simulink model "YCbCrTesting"  (Simulink 7.7)
settings: Solver=ode45  StartTime=0.0  StopTime=10.0  RelTol=1e-3
undefined symbols (not defined in the file or in its folder): gray, M, N, Rec, SDTV, sz
libraries: vipmisc x22, dspsigops x7, viptransforms x6, viputilities x6, vipconversions x4, dspobslib x4, vipobslib x1, dspsrcs4 x1, vipsnks x1
(part 2 of 2)

== matlab function Decoder/Block Processing/Block iterator/sub-block process/Transform decoder1/Bit Unpack ==
  data: in input double; out output single size=64
function out=bitunpack(in)

% Unpack the bits packed by the bit pack block. If there are not enough 
% values in the packed stream the rest of the output is filled with zeros.

persistent prev_out;
if isempty(prev_out)
    prev_out = single(zeros(64,1));
end
    out = prev_out;
    cbits= int32(0); 
    inpos=2; 
    Temp = uint32(0); 
    run = uint32(0);
    val = uint32(0);
   
    numcoefs = 64;
    if bitget(in(1),32)%negative
        out(1)=-int32(intmax('uint32')- uint32(in(1))) - int32(1);
    else
        out(1)=int32(in(1));
    end
    
    % ac coefficients
    % 4 bit - run length followed by 8 bit coef value  
    i=2;
    while (i<=numcoefs)   
         
        [flag, cbits, inpos, Temp, run] = getbits(cbits, inpos, Temp, in, run, 4);
        if (~flag) 
            break; 
        end
        if (run == 15), break;   end % end of stream  
        
        [flag, cbits, inpos, Temp, val] = getbits(cbits, inpos, Temp, in, val, 8);
        if (~flag) 
            break; 
        end 
        
        for j= i: min(run+i, numcoefs)    
            out(j) = single(single(val)-128.0);  
        end
        i = i + double(run)+1;
    end

    % when we havent got all coefs in the stream 
    for i=i:numcoefs    
        out(i) = 0;
    end
    prev_out(:)=out;
end

%%=================================================
function [flag, cbitsO, inposO, TempO, valO] = getbits(cbits, inpos, Temp, in, val, bits)

    lval = uint32(0); 
    temp = uint32(0);
    cbitsO = int32(cbits);
    inposO = inpos;
    TempO = uint32(Temp);
    valO = uint32(val);
    inwidth = length(in);
    if (cbitsO < bits)  
        if (inposO > inwidth) 
            flag=0;
            return; 
        end

        lval(:) =  bitshift(TempO, -(32-cbitsO));  
        bits(:) = bits - cbitsO;
        TempO = in(inposO); inposO = inposO +1;  
        lval = bitshift(lval, bits);  
        cbitsO(:) = int32(32);
    end

    temp(:) = bitshift(TempO, -(32-bits));  
    TempO(:) = bitshift(TempO, bits);  
    valO(:) = bitor(lval, temp); 
    cbitsO(:) = cbitsO - bits;

    flag = 1;
end

== matlab function Decoder/Block Processing/Block iterator/sub-block process/Transform decoder2/Bit Unpack ==
  data: in input double; out output single size=64
function out=bitunpack(in)

% Unpack the bits packed by the bit pack block. If there are not enough 
% values in the packed stream the rest of the output is filled with zeros.

persistent prev_out;
if isempty(prev_out)
    prev_out = single(zeros(64,1));
end
    out = prev_out;
    cbits= int32(0); 
    inpos=2; 
    Temp = uint32(0); 
    run = uint32(0);
    val = uint32(0);
   
    numcoefs = 64;
    if bitget(in(1),32)%negative
        out(1)=-int32(intmax('uint32')- uint32(in(1))) - int32(1);
    else
        out(1)=int32(in(1));
    end
    
    % ac coefficients
    % 4 bit - run length followed by 8 bit coef value  
    i=2;
    while (i<=numcoefs)   
         
        [flag, cbits, inpos, Temp, run] = getbits(cbits, inpos, Temp, in, run, 4);
        if (~flag) 
            break; 
        end
        if (run == 15), break;   end % end of stream  
        
        [flag, cbits, inpos, Temp, val] = getbits(cbits, inpos, Temp, in, val, 8);
        if (~flag) 
            break; 
        end 
        
        for j= i: min(run+i, numcoefs)    
            out(j) = single(single(val)-128.0);  
        end
        i = i + double(run)+1;
    end

    % when we havent got all coefs in the stream 
    for i=i:numcoefs    
        out(i) = 0;
    end
    prev_out(:)=out;
end

%%=================================================
function [flag, cbitsO, inposO, TempO, valO] = getbits(cbits, inpos, Temp, in, val, bits)

    lval = uint32(0); 
    temp = uint32(0);
    cbitsO = int32(cbits);
    inposO = inpos;
    TempO = uint32(Temp);
    valO = uint32(val);
    inwidth = length(in);
    if (cbitsO < bits)  
        if (inposO > inwidth) 
            flag=0;
            return; 
        end

        lval(:) =  bitshift(TempO, -(32-cbitsO));  
        bits(:) = bits - cbitsO;
        TempO = in(inposO); inposO = inposO +1;  
        lval = bitshift(lval, bits);  
        cbitsO(:) = int32(32);
    end

    temp(:) = bitshift(TempO, -(32-bits));  
    TempO(:) = bitshift(TempO, bits);  
    valO(:) = bitor(lval, temp); 
    cbitsO(:) = cbitsO - bits;

    flag = 1;
end

== matlab function Encoder/Block Processing/Block iterator/sub-block process/Transform coder1/Bit Pack ==
  data: in input double; out output uint32 size=20
function out=bitpack(in) 

% Pack output bits into given length using run length coding. The first 
% coefficient (DC) is coded using 32 bits. The AC coefficients are run 
% length coded using 4 bits for run and 8 bits for value. The output is uint32.

persistent prev_out;
if isempty(prev_out)
    prev_out = uint32(zeros(20,1));
end
    out=uint32(prev_out);
    % Bit Pack Routine  
    bitpos=int32(0); 
    Temp= uint32(0); 
    run =  uint32(0); 
    outpos = 2; 
    pval=single(0); 
    cval=single(0);
  
    numcoefs = 64;
    
    out1 =  int32(fix(in(1)));
    
    if out1>=-1   
       out(1) = uint32(out1);
    else
       out(1) = uint32(intmax('uint32') - uint32(abs(out1)) +uint32(2));
    end

    % ac coefficients
    % 4 bit - run length followed by 8 bit coef value  
    pval(:) = fix(in(2)+0.5);
    if (pval > 127),  pval(:) = 127; end % saturate  
    if (pval < -128), pval(:) = -128; end

    run(:) = 0;
    for i=(3): numcoefs   
        cval(:) = floor(in(i)+0.5); 
        if (pval == cval && run < 14)  
            run(:)=run(:)+1;
        else  
            [flag, bitpos, out, Temp, outpos] = putbits(bitpos, out, Temp, outpos, run, 4);
            if (~flag) 
                prev_out=out;
                return; 
            end

            if (pval > 127),  pval(:) = 127;  end % saturate  
            if (pval < -128), pval(:) = -128; end
            pval(:) = pval+128; % make positive  

            [flag, bitpos, out, Temp, outpos] = putbits(bitpos, out, Temp, outpos, uint32(pval), 8);
            if (~flag) 
                prev_out=out;
                return; 
            end

            run(:) = 0;
        end
        pval(:) = cval;
    end

    % last coefficient  
    [flag, bitpos, out, Temp, outpos] = putbits(bitpos, out, Temp, outpos, run, 4);
    if (~flag) 
        prev_out=out;
        return; 
    end

    if (pval > 127),  pval(:) = 127;  end % saturate 
    if (pval < -128), pval(:) = -128; end
    pval(:) = pval+128; % make positive 

    [flag, bitpos, out, Temp, outpos] = putbits(bitpos, out, Temp, outpos, pval, 8);
    if (~flag) 
        prev_out=out;
        return; 
    end

    [bitpos, out, Temp, outpos] = flushbits(bitpos, out, Temp, outpos);%#ok
    prev_out=out;
end

%%========================================================================
function [flag, bitposO, outO, TempO, outposO] = putbits(bitpos, out, Temp, outpos, val, bits)
     
    valIn = uint32(val);
    bitsIn=int32(bits);
    bitposO = int32(bitpos);
    outO = uint32(out);
    TempO = uint32(Temp);
    outposO = outpos;
    
    if (bitposO + bitsIn > 32)  
        bitsleft = int32(32 - bitposO);
        bval=uint32(0);
        bval(:) = bitshift(valIn, -(bitsIn-bitsleft)); 
        TempO(:) = bitor(TempO,bval); 
        outO(outposO) = TempO;
        outposO = outposO+1;
        if (outposO > length(out))  
            flag = 0;
            return;
        end
        TempO = uint32(0);
        bitposO(:) = int32(0);
        bitsIn(:) = bitsIn-bitsleft; 
        valIn(:)=bitshift(valIn, 32-bitsIn);  
        valIn(:)=bitshift(valIn, -(32-bitsIn)); 
    end
    valIn(:)=bitshift(valIn, (32-(bitsIn+(bitposO))));  
    TempO = bitor(TempO, valIn); 
    bitposO(:) = bitposO + bitsIn;
    flag=1;
end

%%========================================================================
function [bitposO, outO, TempO, outposO, out] = flushbits(bitpos, out, Temp, outpos)
 
    [flag, bitposO, outO, TempO, outposO] = putbits(bitpos, out, Temp, outpos, 15, 4);
    if (~flag) 
        return; 
    end
    if (outposO > length(out)+1), return; end
    outO(outposO) = TempO;
end

== matlab function Encoder/Block Processing/Block iterator/sub-block process/Transform coder2/Bit Pack ==
  data: in input double; out output uint32 size=20
function out=bitpack(in) 

% Pack output bits into given length using run length coding. The first 
% coefficient (DC) is coded using 32 bits. The AC coefficients are run 
% length coded using 4 bits for run and 8 bits for value. The output is uint32.

persistent prev_out;
if isempty(prev_out)
    prev_out = uint32(zeros(20,1));
end
    out=uint32(prev_out);
    % Bit Pack Routine  
    bitpos=int32(0); 
    Temp= uint32(0); 
    run =  uint32(0); 
    outpos = 2; 
    pval=single(0); 
    cval=single(0);
  
    numcoefs = 64;
    
    out1 =  int32(fix(in(1)));
    
    if out1>=-1   
       out(1) = uint32(out1);
    else
       out(1) = uint32(intmax('uint32') - uint32(abs(out1)) +uint32(2));
    end

    % ac coefficients
    % 4 bit - run length followed by 8 bit coef value  
    pval(:) = fix(in(2)+0.5);
    if (pval > 127),  pval(:) = 127; end % saturate  
    if (pval < -128), pval(:) = -128; end

    run(:) = 0;
    for i=(3): numcoefs   
        cval(:) = floor(in(i)+0.5); 
        if (pval == cval && run < 14)  
            run(:)=run(:)+1;
        else  
            [flag, bitpos, out, Temp, outpos] = putbits(bitpos, out, Temp, outpos, run, 4);
            if (~flag) 
                prev_out=out;
                return; 
            end

            if (pval > 127),  pval(:) = 127;  end % saturate  
            if (pval < -128), pval(:) = -128; end
            pval(:) = pval+128; % make positive  

            [flag, bitpos, out, Temp, outpos] = putbits(bitpos, out, Temp, outpos, uint32(pval), 8);
            if (~flag) 
                prev_out=out;
                return; 
            end

            run(:) = 0;
        end
        pval(:) = cval;
    end

    % last coefficient  
    [flag, bitpos, out, Temp, outpos] = putbits(bitpos, out, Temp, outpos, run, 4);
    if (~flag) 
        prev_out=out;
        return; 
    end

    if (pval > 127),  pval(:) = 127;  end % saturate 
    if (pval < -128), pval(:) = -128; end
    pval(:) = pval+128; % make positive 

    [flag, bitpos, out, Temp, outpos] = putbits(bitpos, out, Temp, outpos, pval, 8);
    if (~flag) 
        prev_out=out;
        return; 
    end

    [bitpos, out, Temp, outpos] = flushbits(bitpos, out, Temp, outpos);%#ok
    prev_out=out;
end

%%========================================================================
function [flag, bitposO, outO, TempO, outposO] = putbits(bitpos, out, Temp, outpos, val, bits)
     
    valIn = uint32(val);
    bitsIn=int32(bits);
    bitposO = int32(bitpos);
    outO = uint32(out);
    TempO = uint32(Temp);
    outposO = outpos;
    
    if (bitposO + bitsIn > 32)  
        bitsleft = int32(32 - bitposO);
        bval=uint32(0);
        bval(:) = bitshift(valIn, -(bitsIn-bitsleft)); 
        TempO(:) = bitor(TempO,bval); 
        outO(outposO) = TempO;
        outposO = outposO+1;
        if (outposO > length(out))  
            flag = 0;
            return;
        end
        TempO = uint32(0);
        bitposO(:) = int32(0);
        bitsIn(:) = bitsIn-bitsleft; 
        valIn(:)=bitshift(valIn, 32-bitsIn);  
        valIn(:)=bitshift(valIn, -(32-bitsIn)); 
    end
    valIn(:)=bitshift(valIn, (32-(bitsIn+(bitposO))));  
    TempO = bitor(TempO, valIn); 
    bitposO(:) = bitposO + bitsIn;
    flag=1;
end

%%========================================================================
function [bitposO, outO, TempO, outposO, out] = flushbits(bitpos, out, Temp, outpos)
 
    [flag, bitposO, outO, TempO, outposO] = putbits(bitpos, out, Temp, outpos, 15, 4);
    if (~flag) 
        return; 
    end
    if (outposO > length(out)+1), return; end
    outO(outposO) = TempO;
end
